simulink model "backstepping_controller"  (R2021a)
settings: Solver=VariableStepAuto  StartTime=0.0  StopTime=10.0  RelTol=1e-3
libraries: pid_lib x2
settings Model: Creator=dabc  LastModifiedBy=dabc

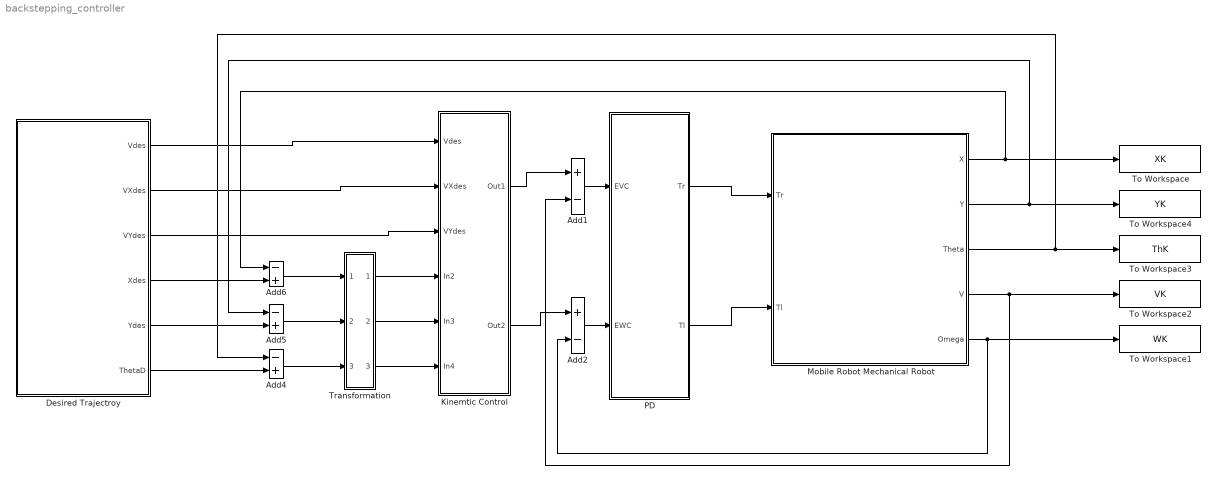
== system backstepping_controller ==
  Add1 : Sum  Inputs=+-
  Add2 : Sum  Inputs=+-
  Add4 : Sum  Inputs=-+
  Add5 : Sum  Inputs=-+
  Add6 : Sum  Inputs=-+
  Desired Trajectroy : Subsystem
  Kinemtic Control : Subsystem
  Mobile Robot Mechanical Robot : Subsystem
  PD : Subsystem
  To Workspace : ToWorkspace  VariableName=XK  SaveFormat=Timeseries  SampleTime=-1
  To Workspace1 : ToWorkspace  VariableName=WK  SaveFormat=Timeseries  SampleTime=-1
  To Workspace2 : ToWorkspace  VariableName=VK  SaveFormat=Timeseries  SampleTime=-1
  To Workspace3 : ToWorkspace  VariableName=ThK  SaveFormat=Timeseries  SampleTime=-1
  To Workspace4 : ToWorkspace  VariableName=YK  SaveFormat=Timeseries  SampleTime=-1
  Transformation : Subsystem
  wires:
  Mobile Robot Mechanical Robot/1(X) -> To Workspace/1, Add6/1
  Mobile Robot Mechanical Robot/2(Y) -> Add5/1, To Workspace4/1
  Transformation/1(Out1) -> Kinemtic Control/4(In2)
  Transformation/2(Out2) -> Kinemtic Control/5(In3)
  Transformation/3(Out3) -> Kinemtic Control/6(In4)
  Desired Trajectroy/1(Vdes) -> Kinemtic Control/1(Vdes)
  Desired Trajectroy/2(VXdes) -> Kinemtic Control/2(VXdes)
  Desired Trajectroy/3(VYdes) -> Kinemtic Control/3(VYdes)
  Add6/1 -> Transformation/1(In1)
  Add5/1 -> Transformation/2(In2)
  Add4/1 -> Transformation/3(In3)
  Desired Trajectroy/4(Xdes) -> Add6/2
  Desired Trajectroy/5(Ydes) -> Add5/2
  Desired Trajectroy/6(ThetaD) -> Add4/2
  Mobile Robot Mechanical Robot/3(Theta) -> To Workspace3/1, Add4/1
  Mobile Robot Mechanical Robot/4(V) -> To Workspace2/1, Add1/2
  Mobile Robot Mechanical Robot/5(Omega) -> Add2/2, To Workspace1/1
  Add2/1 -> PD/2(EWC)
  Add1/1 -> PD/1(EVC)
  Kinemtic Control/1(Out1) -> Add1/1
  Kinemtic Control/2(Out2) -> Add2/1
  PD/1(Tr) -> Mobile Robot Mechanical Robot/1(Tr)
  PD/2(Tl) -> Mobile Robot Mechanical Robot/2(Tl)

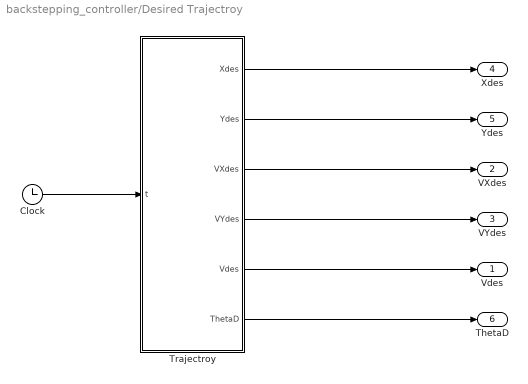
== system backstepping_controller/Desired Trajectroy ==
  Clock : Clock
  Trajectroy : MATLAB Function  TreatAsAtomicUnit=on
  Vdes : Outport
  VXdes : Outport  Port=2
  VYdes : Outport  Port=3
  Xdes : Outport  Port=4
  Ydes : Outport  Port=5
  ThetaD : Outport  Port=6
  wires:
  Clock/1 -> Trajectroy/1(t)
  Trajectroy/1(Xdes) -> Xdes/1
  Trajectroy/2(Ydes) -> Ydes/1
  Trajectroy/3(VXdes) -> VXdes/1
  Trajectroy/4(VYdes) -> VYdes/1
  Trajectroy/5(Vdes) -> Vdes/1
  Trajectroy/6(ThetaD) -> ThetaD/1

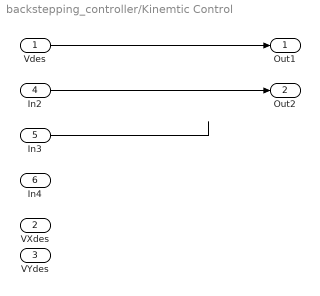
== system backstepping_controller/Kinemtic Control ==
  Vdes : Inport
  VXdes : Inport  Port=2
  VYdes : Inport  Port=3
  In2 : Inport  Port=4
  In3 : Inport  Port=5
  In4 : Inport  Port=6
  Out1 : Outport
  Out2 : Outport  Port=2
  wires:
  Vdes/1 -> Out1/1
  In2/1 -> Out2/1
  In3/1 -> ?

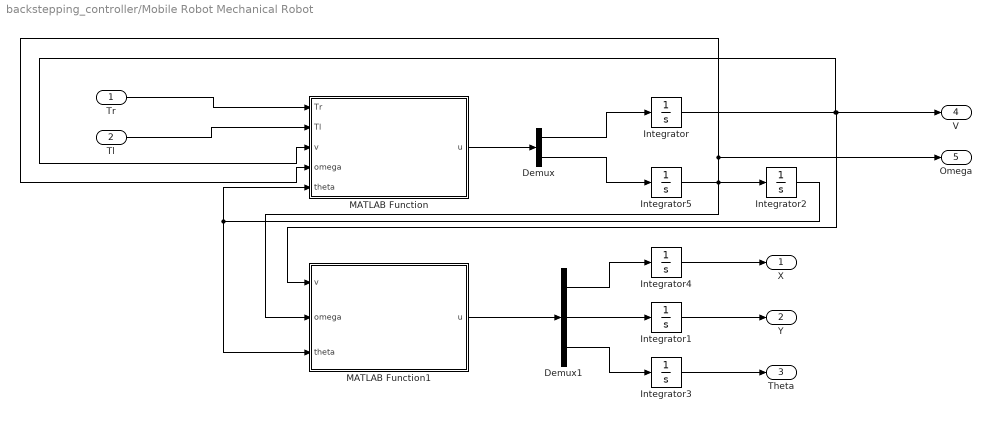
== system backstepping_controller/Mobile Robot Mechanical Robot ==
  Tr : Inport  OutMin=[0]  OutMax=15
  Tl : Inport  Port=2  OutMin=[0]  OutMax=[15]
  Demux : Demux  Outputs=2
  Demux1 : Demux  Outputs=3
  Integrator{,1..5} (6 alike) : Integrator
  MATLAB Function : MATLAB Function  TreatAsAtomicUnit=on
  MATLAB Function1 : MATLAB Function  TreatAsAtomicUnit=on
  X : Outport
  Y : Outport  Port=2
  Theta : Outport  Port=3
  V : Outport  Port=4
  Omega : Outport  Port=5
  wires:
  Demux1/2 -> Integrator1/1
  MATLAB Function/1(u) -> Demux/1
  Demux1/1 -> Integrator4/1
  Integrator5/1 -> MATLAB Function1/2(omega), Integrator2/1, Omega/1, MATLAB Function/4(omega)
  Integrator2/1 -> MATLAB Function1/3(theta), MATLAB Function/5(theta)
  Tl/1 -> MATLAB Function/2(Tl)
  Integrator/1 -> MATLAB Function/3(v), MATLAB Function1/1(v), V/1
  Integrator1/1 -> Y/1
  MATLAB Function1/1(u) -> Demux1/1
  Integrator3/1 -> Theta/1
  Demux/2 -> Integrator5/1
  Integrator4/1 -> X/1
  Demux/1 -> Integrator/1
  Tr/1 -> MATLAB Function/1(Tr)
  Demux1/3 -> Integrator3/1

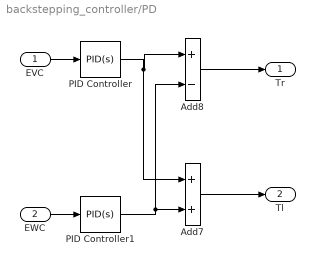
== system backstepping_controller/PD ==
  EVC : Inport
  EWC : Inport  Port=2
  Add7 : Sum
  Add8 : Sum  Inputs=+-
  PID Controller : pid_lib/PID Controller  Controller=PID  Form=Parallel  TimeDomain=Continuous-time  UseExternalTs=off  SampleTime=-1  IntegratorMethod=Forward Euler  FilterMethod=Forward Euler  ControllerParametersSource=internal  P=1  I=1  D=0  UseFilter=on  N=100  TunerSelectOption=Transfer Function Based (PID Tuner App)  InitialConditionSource=internal  InitialConditionForIntegrator=0  InitialConditionForFilter=0  DifferentiatorICPrevScaledInput=0  ExternalReset=none  TrackingMode=off  Kt=1  LimitOutput=off  SatLimitsSource=internal  UpperSaturationLimit=inf  LowerSaturationLimit=-inf  LinearizeAsGain=on  AntiWindupMode=none  Kb=1  POutMin=[]  POutMax=[]  IOutMin=[]  IOutMax=[]  DOutMin=[]  DOutMax=[]  NOutMin=[]  NOutMax=[]  SumOutMin=[]  SumOutMax=[]  SaturationOutMin=[]  SaturationOutMax=[]  PParamMin=[]  PParamMax=[]  IParamMin=[]  IParamMax=[]  DParamMin=[]  DParamMax=[]  NParamMin=[]  NParamMax=[]  KbParamMin=[]  KbParamMax=[]  KtParamMin=[]  KtParamMax=[]  KbOutMin=[]  KbOutMax=[]  KtOutMin=[]  KtOutMax=[]  IntegratorOutMin=[]  IntegratorOutMax=[]  FilterOutMin=[]  FilterOutMax=[]  SumI1OutMin=[]  SumI1OutMax=[]  SumI2OutMin=[]  SumI2OutMax=[]  SumI3OutMin=[]  SumI3OutMax=[]  SumI4OutMin=[]  SumI4OutMax=[]  SumDOutMin=[]  SumDOutMax=[]  DifferentiatorOutMin=[]  DifferentiatorOutMax=[]  FilterDiffOutCoefMin=[]  FilterDiffOutCoefMax=[]  ReciprocalOutMin=[]  ReciprocalOutMax=[]  SumDenOutMin=[]  SumDenOutMax=[]  SumNumOutMin=[]  SumNumOutMax=[]  DivideOutMin=[]  DivideOutMax=[]  UdiffTsProdOutMin=[]  UdiffTsProdOutMax=[]  NTsProdOutMin=[]  NTsProdOutMax=[]  UintegralTsProdOutMin=[]  UintegralTsProdOutMax=[]  UngainTsProdOutMin=[]  UngainTsProdOutMax=[]  IntegratorContinuousStateAttributes=''  IntegratorStateMustResolveToSignalObject=off  IntegratorRTWStateStorageClass=Auto  FilterContinuousStateAttributes=''  FilterStateMustResolveToSignalObject=off  FilterRTWStateStorageClass=Auto  ParallelPVariant=InternalParameters  IdealPVariant=Disabled  IVariant=InternalParameters  DVariant=InternalParameters  IntegratorVariant=Continuous  SatVariant=Disabled  AWVariant=Passthrough  PCopyVariant=Disabled  TRVariant=Disabled  FdbkBlocksVariant=Forward  IdealPFdbkVariant=Disabled  SatFdbkVariant=Disabled  DerivativeFilterVariant=ContFilter  NVariant=InternalParameters  NCopyVariant=Disabled  FilterICVariant=InternalICsFilter  IntegratorICVariant=InternalICs  ExternalResetVariant=Disabled  TRSumVariant=Passthrough  SumFdbkVariant=Disabled  SumVariant=Sum_PID  TsampFilterVariant=InternalTs  TsampNgainVariant=Passthrough  TsampIntegralVariant=Passthrough  ExternalSaturationOutDataTypeStr=Inherit: Same as second input
  PID Controller1 : pid_lib/PID Controller  Controller=PID  Form=Parallel  TimeDomain=Continuous-time  UseExternalTs=off  SampleTime=-1  IntegratorMethod=Forward Euler  FilterMethod=Forward Euler  ControllerParametersSource=internal  P=1  I=1  D=0  UseFilter=on  N=100  TunerSelectOption=Transfer Function Based (PID Tuner App)  InitialConditionSource=internal  InitialConditionForIntegrator=0  InitialConditionForFilter=0  DifferentiatorICPrevScaledInput=0  ExternalReset=none  TrackingMode=off  Kt=1  LimitOutput=off  SatLimitsSource=internal  UpperSaturationLimit=inf  LowerSaturationLimit=-inf  LinearizeAsGain=on  AntiWindupMode=none  Kb=1  POutMin=[]  POutMax=[]  IOutMin=[]  IOutMax=[]  DOutMin=[]  DOutMax=[]  NOutMin=[]  NOutMax=[]  SumOutMin=[]  SumOutMax=[]  SaturationOutMin=[]  SaturationOutMax=[]  PParamMin=[]  PParamMax=[]  IParamMin=[]  IParamMax=[]  DParamMin=[]  DParamMax=[]  NParamMin=[]  NParamMax=[]  KbParamMin=[]  KbParamMax=[]  KtParamMin=[]  KtParamMax=[]  KbOutMin=[]  KbOutMax=[]  KtOutMin=[]  KtOutMax=[]  IntegratorOutMin=[]  IntegratorOutMax=[]  FilterOutMin=[]  FilterOutMax=[]  SumI1OutMin=[]  SumI1OutMax=[]  SumI2OutMin=[]  SumI2OutMax=[]  SumI3OutMin=[]  SumI3OutMax=[]  SumI4OutMin=[]  SumI4OutMax=[]  SumDOutMin=[]  SumDOutMax=[]  DifferentiatorOutMin=[]  DifferentiatorOutMax=[]  FilterDiffOutCoefMin=[]  FilterDiffOutCoefMax=[]  ReciprocalOutMin=[]  ReciprocalOutMax=[]  SumDenOutMin=[]  SumDenOutMax=[]  SumNumOutMin=[]  SumNumOutMax=[]  DivideOutMin=[]  DivideOutMax=[]  UdiffTsProdOutMin=[]  UdiffTsProdOutMax=[]  NTsProdOutMin=[]  NTsProdOutMax=[]  UintegralTsProdOutMin=[]  UintegralTsProdOutMax=[]  UngainTsProdOutMin=[]  UngainTsProdOutMax=[]  IntegratorContinuousStateAttributes=''  IntegratorStateMustResolveToSignalObject=off  IntegratorRTWStateStorageClass=Auto  FilterContinuousStateAttributes=''  FilterStateMustResolveToSignalObject=off  FilterRTWStateStorageClass=Auto  ParallelPVariant=InternalParameters  IdealPVariant=Disabled  IVariant=InternalParameters  DVariant=InternalParameters  IntegratorVariant=Continuous  SatVariant=Disabled  AWVariant=Passthrough  PCopyVariant=Disabled  TRVariant=Disabled  FdbkBlocksVariant=Forward  IdealPFdbkVariant=Disabled  SatFdbkVariant=Disabled  DerivativeFilterVariant=ContFilter  NVariant=InternalParameters  NCopyVariant=Disabled  FilterICVariant=InternalICsFilter  IntegratorICVariant=InternalICs  ExternalResetVariant=Disabled  TRSumVariant=Passthrough  SumFdbkVariant=Disabled  SumVariant=Sum_PID  TsampFilterVariant=InternalTs  TsampNgainVariant=Passthrough  TsampIntegralVariant=Passthrough  ExternalSaturationOutDataTypeStr=Inherit: Same as second input
  Tr : Outport
  Tl : Outport  Port=2
  wires:
  PID Controller/1 -> Add7/1, Add8/1
  EVC/1 -> PID Controller/1
  Add8/1 -> Tr/1
  PID Controller1/1 -> Add8/2, Add7/2
  EWC/1 -> PID Controller1/1
  Add7/1 -> Tl/1

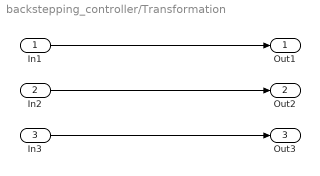
== system backstepping_controller/Transformation ==
  In1 : Inport
  In2 : Inport  Port=2
  In3 : Inport  Port=3
  Out1 : Outport
  Out2 : Outport  Port=2
  Out3 : Outport  Port=3
  wires:
  In1/1 -> Out1/1
  In2/1 -> Out2/1
  In3/1 -> Out3/1

== matlab function backstepping_controller/Mobile Robot Mechanical Robot/MATLAB Function ==
  data: Tr input; u output; Tl input; v input; omega input; theta input
function u=Dynamics(Tr,Tl,v,omega,theta) 
m=10;           
Ra=0.05;        
a=0.05;         
axis 
L = 0.5;        
J=5;            
% The robot mass 
% The radius of the wheels 
% The distance between the center of mass and wheels 
% The lateral distance of the wheels to the center 
% The robot mass moment of inertia 
M=[m 0 m*a*sin(theta); 
    0 m -m*a*cos(theta); 
    m*a*sin(theta) -m*a*cos(theta) J]; 
V=[0 0 m*a*omega*cos(theta); 
    0 0 m*a*omega*sin(theta) 
    0 0 0]; 
S=[cos(theta) -a*sin(theta); 
    sin(theta) a*cos(theta); 
    0 1]; 
B=[cos(theta)/Ra cos(theta)/Ra; 
    sin(theta)/Ra sin(theta)/Ra; 
    L/Ra -L/Ra]; 
Sdot=[-omega*sin(theta) -a*omega*cos(theta); 
      omega*cos(theta)   -a*omega*sin(theta); 
      0 0]; 
Mh=S'*M*S; 
Vh=[0 -m*a*omega; 
     m*a*omega 0]; 
Bh=S'*B; 
T=[Tr;Tl]; 
ve=[v;omega]; 
vdot=inv(Mh)*(T-Vh*ve); 
u=[vdot(1),vdot(2)];

== matlab function backstepping_controller/Desired Trajectroy/Trajectroy ==
  data: t input; Xdes output; Ydes output; VXdes output; VYdes output; Vdes output; ThetaD output
function [Xdes, Ydes, VXdes, VYdes, Vdes, ThetaD] = Trajectory(t)
    % t: الوقت الحالي المُدخل من الـClock

    % تحديد المسار المطلوب (على سبيل المثال، مسار دائري)
    R = 5; % نصف قطر الدائرة
    omega = 0.1; % السرعة الزاوية (rad/s)

    % حساب القيم المرجعية بناءً على الزمن الحالي t
    Xdes = R * cos(omega * t); % الموقع المطلوب على المحور X
    Ydes = R * sin(omega * t); % الموقع المطلوب على المحور Y

    % حساب السرعة المطلوبة
    VXdes = -R * omega * sin(omega * t); % السرعة المطلوبة على المحور X
    VYdes = R * omega * cos(omega * t);  % السرعة المطلوبة على المحور Y

    % حساب السرعة الخطية المطلوبة
    Vdes = sqrt(VXdes^2 + VYdes^2); % السرعة الخطية

    % حساب الزاوية المطلوبة (الاتجاه)
    ThetaD = atan2(VYdes, VXdes); % الزاوية المطلوبة

end

== matlab function backstepping_controller/Mobile Robot Mechanical Robot/MATLAB Function1 ==
  data: v input; u output; omega input; theta input
function u=Kinematics(v,omega,theta) 
m=10; 
Ra=0.05; 
a=0.05; 
L = 0.5; 
J=5; 
S=[cos(theta) -a*sin(theta); 
    sin(theta) a*cos(theta); 
    0 1]; 
ve=[v;omega]; 
qdot=S*ve; 
u=[qdot(1),qdot(2),qdot(3)];
